simulink model "AsteroidImpact"  (R2021b)
settings: Solver=ode4  StartTime=0.0  StopTime=45  FixedStep=0.1  RelTol=1e-3
libraries: cstblocks x1, dspsigops x1
settings Model: Creator=KNMALE002  LastModifiedBy=lbaat
settings SolverCC: AlgebraicLoopSolver=TrustRegion
settings DataIOCC: SaveOutput=off  SignalLogging=off  DSMLogging=off  ReturnWorkspaceOutputs=off  TimeSaveName=simulation_time
settings DebuggingCC: SFMachineParentedDataDiag=warning  ArithmeticOperatorsInVariantConditions=warning
settings SFSimCC: CustomCodeUndefinedFunction=UseInterfaceOnly

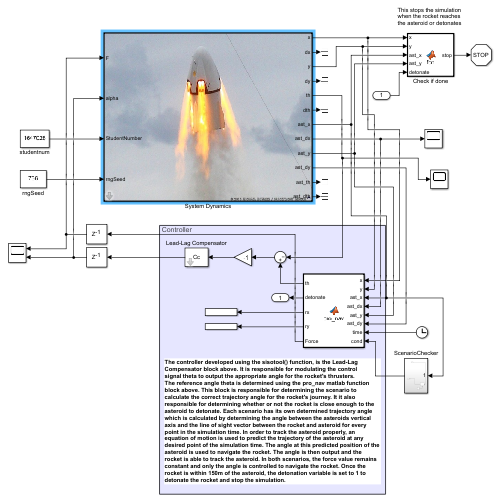
[thumbnail: Simulink's stored preview of the top-level diagram]
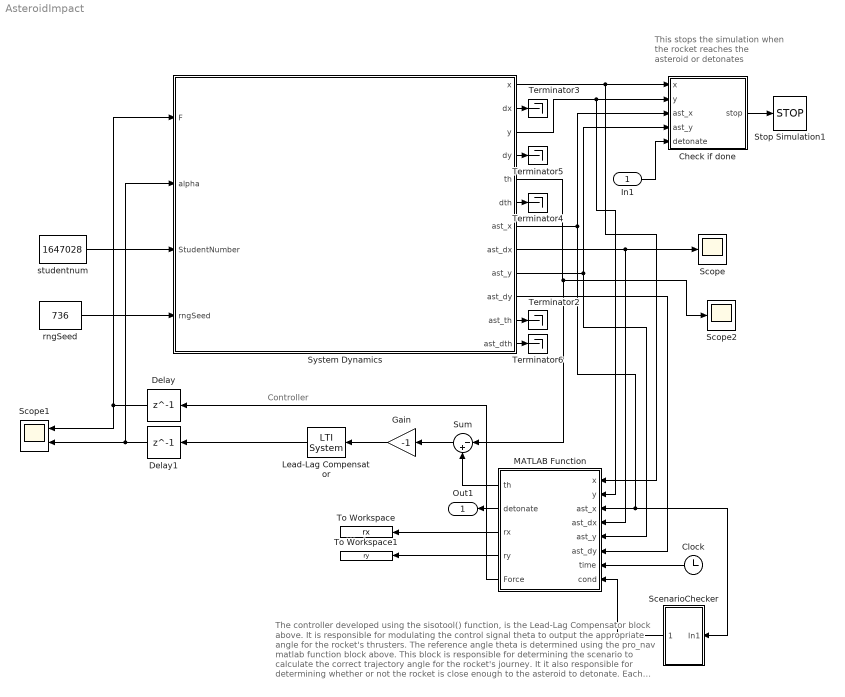
== system AsteroidImpact ==
  note: The controller developed using the sisotool() function, is the Lead-Lag Compensator block above. It is responsible for modulating the control
      | signal theta to output the appropriate angle for the rocket's thrusters.
      | The reference angle theta is determined using the pro_nav matlab function
      | block above. This block is responsible for determining the scenario to
      | calculate the correct trajectory angle for the rocket's journey. It it also
      | responsible for determining whether or not the rocket is close enough to the asteroid to detonate. Each scenario has its own determined trajectory angle
      | which is calculated by determining the angle between the asteroids vertical
      | axis and the line of sight vector between the rocket and asteroid for every point in the simulation time. In order to track the asteroid properly, an equation of motion is used to predict the trajectory of the asteroid at any desired point of the simulation time. The angle at this predicted position of the asteroid is used to navigate the rocket. The angle is then output and the rocket is able to track the asteroid. In both scenarios, the force value remains constant and only the angle is controlled to navigate the rocket. Once the rocket is within 150m of the asteroid, the detonation variable is set to 1 to detonate the rocket and stop the simulation.
  note: Controller
  note: This stops the simulation when the rocket reaches the asteroid or detonates
  In1 : Inport
  Check if done : MATLAB Function  TreatAsAtomicUnit=on
  Clock : Clock
  Delay : Delay  DelayLength=1  InitialCondition=10000000000
  Delay1 : Delay  DelayLength=1
  Gain : Gain  Gain=-1
  Lead-Lag Compensator : cstblocks/LTI System  sys=Cc  IC=[]
  MATLAB Function : MATLAB Function  TreatAsAtomicUnit=on
  ScenarioChecker : Subsystem
  Scope : Scope
  Scope1 : Scope  NumInputPorts=2
  Scope2 : Scope
  Stop Simulation1 : Stop
  Sum : Sum  Inputs=|-+
  System Dynamics : Subsystem  TreatAsAtomicUnit=on  mask{Value=1}
      mask prompts: Value "Enter mode (1, 2 or 3)"
      mask TypeOptions Value: ScenarioVar/Value
      mask Display: image('lander.jpg');
  Terminator{2..6} (5 alike) : Terminator
  To Workspace : ToWorkspace  VariableName=rx  SaveFormat=Structure With Time  SampleTime=-1
  To Workspace1 : ToWorkspace  VariableName=ry  SaveFormat=Structure With Time  SampleTime=-1
  rngSeed : Constant  Value=736
  studentnum : Constant  Value=1647028
  Out1 : Outport
  wires:
  studentnum/1 -> System Dynamics/3(StudentNumber)
  System Dynamics/1(x) -> MATLAB Function/1(x), Check if done/1(x)
  rngSeed/1 -> System Dynamics/4(rngSeed)
  System Dynamics/3(y) -> MATLAB Function/2(y), Check if done/2(y)
  System Dynamics/12(ast_dth) -> Terminator6/1
  System Dynamics/7(ast_x) -> ScenarioChecker/1(In1), MATLAB Function/3(ast_x), Check if done/3(ast_x)
  System Dynamics/9(ast_y) -> MATLAB Function/5(ast_y), Check if done/4(ast_y)
  System Dynamics/8(ast_dx) -> MATLAB Function/4(ast_dx), Scope/1
  Check if done/1(stop) -> Stop Simulation1/1
  Delay1/1 -> System Dynamics/2(alpha), Scope1/2
  In1/1 -> Check if done/5(detonate)
  System Dynamics/10(ast_dy) -> MATLAB Function/6(ast_dy)
  System Dynamics/2(dx) -> Terminator3/1
  System Dynamics/6(dth) -> Terminator4/1
  System Dynamics/4(dy) -> Terminator5/1
  System Dynamics/5(th) -> Sum/1, Scope2/1
  Delay/1 -> System Dynamics/1(F), Scope1/1
  Sum/1 -> Gain/1
  Gain/1 -> Lead-Lag Compensator/1
  Lead-Lag Compensator/1 -> Delay1/1
  Clock/1 -> MATLAB Function/7(time)
  MATLAB Function/2(detonate) -> Out1/1
  MATLAB Function/3(rx) -> To Workspace/1
  MATLAB Function/4(ry) -> To Workspace1/1
  MATLAB Function/5(Force) -> Delay/1
  MATLAB Function/1(th) -> Sum/2
  System Dynamics/11(ast_th) -> Terminator2/1
  ScenarioChecker/1(" ") -> MATLAB Function/8(cond)

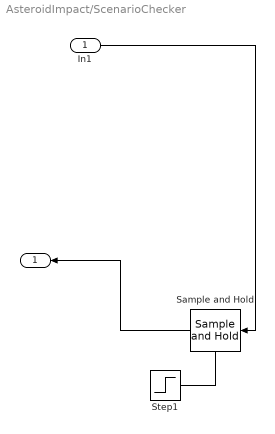
== system AsteroidImpact/ScenarioChecker ==
  In1 : Inport
  Sample and Hold : dspsigops/Sample and Hold  trig=Rising edge  initCond=0  latchinput=on
  Step1 : Step  Time=0.01  SampleTime=0.2
  " " : Outport
  wires:
  Step1/1 -> Sample and Hold/Trigger
  Sample and Hold/1 -> " "/1
  In1/1 -> Sample and Hold/1

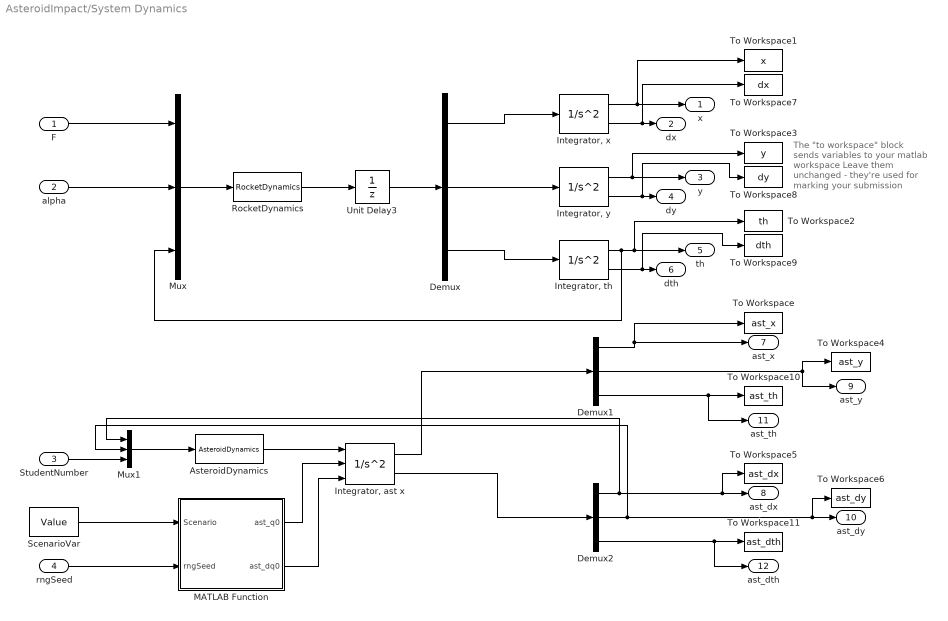
== system AsteroidImpact/System Dynamics ==
  note: The "to workspace" block sends variables to your matlab workspace
      |
      | Leave them unchanged - they're used for marking your submission
  F : Inport
  alpha : Inport  Port=2
  StudentNumber : Inport  Port=3
  rngSeed : Inport  Port=4
  AsteroidDynamics : MATLABFcn  MATLABFcn=AsteroidDynamics  OutputDimensions=3
  Demux : Demux  Outputs=3
  Demux1 : Demux  Outputs=3
  Demux2 : Demux  Outputs=3
  "Integrator, th" : SecondOrderIntegrator  ICX=0  ICDXDT=0
  "Integrator, x" : SecondOrderIntegrator  ICX=0
  "Integrator, y" : SecondOrderIntegrator  ICX=0
  "Integrator, ast x" : SecondOrderIntegrator  ICSourceX=external  ICX=x0  ICSourceDXDT=external
  MATLAB Function : MATLAB Function  TreatAsAtomicUnit=on
  Mux : Mux  Inputs=3
  Mux1 : Mux  Inputs=3
  RocketDynamics : MATLABFcn  MATLABFcn=RocketDynamics  Output1D=off
  ScenarioVar : Constant  Value=Value
  To Workspace : ToWorkspace  VariableName=ast_x  SampleTime=-1
  To Workspace1 : ToWorkspace  VariableName=x  SampleTime=-1
  To Workspace10 : ToWorkspace  VariableName=ast_th  SampleTime=-1
  To Workspace11 : ToWorkspace  VariableName=ast_dth  SampleTime=-1
  To Workspace2 : ToWorkspace  VariableName=th  SampleTime=-1
  To Workspace3 : ToWorkspace  VariableName=y  SampleTime=-1
  To Workspace4 : ToWorkspace  VariableName=ast_y  SampleTime=-1
  To Workspace5 : ToWorkspace  VariableName=ast_dx  SampleTime=-1
  To Workspace6 : ToWorkspace  VariableName=ast_dy  SampleTime=-1
  To Workspace7 : ToWorkspace  VariableName=dx  SampleTime=-1
  To Workspace8 : ToWorkspace  VariableName=dy  SampleTime=-1
  To Workspace9 : ToWorkspace  VariableName=dth  SampleTime=-1
  Unit Delay3 : UnitDelay  SampleTime=-1  HasFrameUpgradeWarning=on
  x : Outport  PortDimensions=1  VectorParamsAs1DForOutWhenUnconnected=off
  dx : Outport  Port=2  PortDimensions=1  VectorParamsAs1DForOutWhenUnconnected=off
  y : Outport  Port=3  PortDimensions=1  VectorParamsAs1DForOutWhenUnconnected=off
  dy : Outport  Port=4  PortDimensions=1  VectorParamsAs1DForOutWhenUnconnected=off
  th : Outport  Port=5  PortDimensions=1  VectorParamsAs1DForOutWhenUnconnected=off
  dth : Outport  Port=6  PortDimensions=1  VectorParamsAs1DForOutWhenUnconnected=off
  ast_x : Outport  Port=7  PortDimensions=1  VectorParamsAs1DForOutWhenUnconnected=off
  ast_dx : Outport  Port=8  PortDimensions=1  VectorParamsAs1DForOutWhenUnconnected=off
  ast_y : Outport  Port=9  PortDimensions=1  VectorParamsAs1DForOutWhenUnconnected=off
  ast_dy : Outport  Port=10  PortDimensions=1  VectorParamsAs1DForOutWhenUnconnected=off
  ast_th : Outport  Port=11  PortDimensions=1  VectorParamsAs1DForOutWhenUnconnected=off
  ast_dth : Outport  Port=12  PortDimensions=1  VectorParamsAs1DForOutWhenUnconnected=off
  wires:
  "Integrator, th"/1 -> Mux/3, th/1, To Workspace2/1
  Demux/1 -> "Integrator, x"/1
  Demux/2 -> "Integrator, y"/1
  Demux/3 -> "Integrator, th"/1
  "Integrator, x"/1 -> x/1, To Workspace1/1
  "Integrator, x"/2 -> To Workspace7/1, dx/1
  "Integrator, y"/2 -> To Workspace8/1, dy/1
  "Integrator, th"/2 -> To Workspace9/1, dth/1
  Mux/1 -> RocketDynamics/1
  RocketDynamics/1 -> Unit Delay3/1
  rngSeed/1 -> MATLAB Function/2(rngSeed)
  ScenarioVar/1 -> MATLAB Function/1(Scenario)
  F/1 -> Mux/1
  alpha/1 -> Mux/2
  Demux1/2 -> To Workspace4/1, ast_y/1
  Demux1/3 -> To Workspace10/1, ast_th/1
  Demux2/3 -> ast_dth/1, To Workspace11/1
  Mux1/1 -> AsteroidDynamics/1
  AsteroidDynamics/1 -> "Integrator, ast x"/1
  "Integrator, ast x"/1 -> Demux1/1
  "Integrator, ast x"/2 -> Demux2/1
  Demux1/1 -> To Workspace/1, ast_x/1
  Demux2/1 -> Mux1/1, To Workspace5/1, ast_dx/1
  Demux2/2 -> Mux1/2, To Workspace6/1, ast_dy/1
  MATLAB Function/1(ast_q0) -> "Integrator, ast x"/2
  MATLAB Function/2(ast_dq0) -> "Integrator, ast x"/3
  StudentNumber/1 -> Mux1/3
  Unit Delay3/1 -> Demux/1
  "Integrator, y"/1 -> y/1, To Workspace3/1

== matlab function AsteroidImpact/System Dynamics/MATLAB Function ==
  data: ast_q0 output; ast_dq0 output; Scenario input; rngSeed input
function [ast_q0, ast_dq0] = fcn(Scenario, rngSeed)
rng(rngSeed);

if (Scenario == 1)
    x0 = -3000;
    y0 =  5000;
    th0 =   0;
    dx0 = 182;
    dy0 = 0;
    dth0 = 0;

elseif (Scenario == 2)
    x0 = -2000 + rand_within_plus_minus(100);
    y0 = 4000 + rand_within_plus_minus(100); 
    th0 = 0;
    dx0 = 170;
    dy0 = 0;
    dth0 = 0.1;

elseif (Scenario == 3)
    x0 = -2500;
    y0 = 3000;
    th0 = 0;
    dx0 = 160;
    dy0 = 100;
    dth0 = deg2rad(rand_within_plus_minus(20)); % rad/sec

else
    error('You entered an invalid mode -- make sure Scenario = 1, 2 or 3')
end

ast_q0  = [ x0;  y0;  th0];
ast_dq0 = [dx0; dy0; dth0];

end

% calling rand_within_plus_minus(100) returns a number between -100 and 100
function n = rand_within_plus_minus(interval)
    n = (rand - 0.5) * 2 * interval;
end

== matlab function AsteroidImpact/MATLAB Function ==
  data: x input; th output; y input; ast_x input; ast_dx input; ast_y input; ast_dy input; time input; detonate output; rx output; ry output; cond input; Force output
function [th, detonate, rx, ry, Force] = pro_nav(x, y, ast_x, ast_dx, ast_y, ast_dy, time, cond)

%% _Determine Scenario From Initial Conditions_
%
if (cond == -3000)
    scenario = 1;
else
    scenario = 2;
end

%% _Determine Trajectory_

if scenario == 2
    % _Trajectory Estimation_
    %
    % Using equation of motion to predict position of asteroid after a few increments
    % r = r_0 + V_0*t + 0.5*a*t^2
    
    Force = 29275;
    Ts = 0.1;
    dt = 8*Ts;
    rx = ast_x + ast_dx*(time+dt);
    ry = ast_y + ast_dy*(time+dt) + 0.5*(-9.81)*((time+dt)^2);


    % _PROPORTIONAL NAVIGATION_
    % Track using theta
    dist = (x - rx);

    xrange = x - rx;
    yrange = ry - y;

    % Determine tracking angle based on where (above or below) asteroid is
    if ry > y % Asteroid above rocket

        % Only start tracking after asteroid is close to position directly
        % above rocket
        if dist > 100
            th = pi/39.84;
        else
            th = atan(xrange/yrange);
        end

    else % ASTEROID BELOW ROCKET
        th = -atan(xrange/yrange);
    end

else
    Force = 31825;
    Ts = 0.1;
    dt = 10*Ts;
    rx = ast_x + ast_dx*(time+dt);
    ry = ast_y + ast_dy*(time+dt) + 0.5*(-9.81)*((time+dt)^2);

    dist = (x - rx);
    xrange = x - rx;
    yrange = ry - y;
    
    % Asteroid above rocket
    if ry > y

        % Only start tracking after asteroid is close to position directly
        % above rocket
        if dist > 0
            th = pi/17;
        else
            th = atan(xrange/yrange);
        end

    else % ASTEROID BELOW ROCKET
        th = -atan(xrange/yrange);
    end

end

%% _SET DETONATION_

Xrange = abs(x - ast_x);
Yrange = abs(y - ast_y);
Dist = sqrt((Xrange^2) + (Yrange^2));

if Dist < 150
    detonate = 1;
else
    detonate = 0;
end

%% _OUTPUTS_

out = [th, detonate, rx, ry, Force];

== matlab function AsteroidImpact/Check if done ==
  data: x input; stop output; y input; ast_x input; ast_y input; detonate input
function stop = fcn(x, y, ast_x, ast_y, detonate)
    % given the signal to detonate
    if detonate == 1
        stop = 1;

    % rocket has hit the asteroid
    elseif norm([x; y] - [ast_x; ast_y]) < 100
        stop = 1;
    
    % rocket has hit the ground OR asteroid is close to they city
    elseif y < 0 || ast_y < 200
        stop = 1;
    
    else
        stop = 0;
    end
end
